simulink model "svpwm_V"  (R2023b)
settings: Solver=FixedStepDiscrete  StartTime=0.0  StopTime=0.05  FixedStep=0.001  MaxStep=0.00001  RelTol=1e-3
libraries: simulink x3
settings Model: Creator=Administrator  LastModifiedBy=LQY
settings SolverCC: AlgebraicLoopSolver=TrustRegion
settings DataIOCC: LimitDataPoints=on  SaveFormat=Array  SignalLoggingSaveFormat=ModelDataLogs  ReturnWorkspaceOutputs=off
settings OptimizationCC: DefaultParameterBehavior=Inlined  UseDivisionForNetSlopeComputation=on  GainParamInheritBuiltInType=on  UseFloatMulNetSlope=on  InlineInvariantSignals=on  PassReuseOutputArgsAs=Individual arguments  ExpressionDepthLimit=2147483647  ZeroExternalMemoryAtStartup=off  ZeroInternalMemoryAtStartup=off  NoFixptDivByZeroProtection=on  EfficientFloat2IntCast=on  LifeSpan=1  OptimizeBlockOrder=speed  DifferentSizesBufferReuse=on  EfficientTunableParamExpr=on
settings DebuggingCC: SaveWithParameterizedLinksMsg=none  UnderspecifiedInitializationDetection=Classic  MergeDetectMultiDrivingBlocksExec=none  SignalResolutionControl=TryResolveAllWithWarning  SolverPrmCheckMsg=warning  MultiTaskDSMMsg=warning  MultiTaskCondExecSysMsg=none  ParameterPrecisionLossMsg=none  ParameterTunabilityLossMsg=error  FcnCallInpInsideContextMsg=warning  UnconnectedInputMsg=warning  UnconnectedOutputMsg=warning  UnconnectedLineMsg=warning  StateNameClashWarn=warning  SFUnexpectedBacktrackingDiag=warning  SFNoUnconditionalDefaultTransitionDiag=warning  SFExecutionAtInitializationDiag=none  ArithmeticOperatorsInVariantConditions=warning
settings HardwareCC: ProdLongLongMode=on
settings ModelReferenceCC: PropagateSignalLabelsOutOfModel=off
settings SFSimCC: SimUseLocalCustomCode=off  MATLABDynamicMemAlloc=off  CustomCodeUndefinedFunction=UseInterfaceOnly
settings RTWCC: Description=Embedded Coder  SystemTargetFile=ert.tlc  GenCodeOnly=on  TemplateMakefile=ert_default_tmf  RTWUseLocalCustomCode=off
settings CodeAppCC: ForceParamTrailComments=on  IgnoreCustomStorageClasses=off  OperatorAnnotations=on  SimulinkDataObjDesc=on  SFDataObjDesc=on  CustomSymbolStrGlobalVar=rt$N$M  CustomSymbolStrType=$N$M  CustomSymbolStrFcn=$N$M$F  CustomSymbolStrMacro=$N$M  InsertBlockDesc=on
settings ERTTargetCC: GenerateSampleERTMain=on  IncludeMdlTerminateFcn=off  CombineSignalStateStructs=on  SuppressErrorStatus=on  SupportAbsoluteTime=off  SupportComplex=off  InlinedParameterPlacement=NonHierarchical  ERTCustomFileTemplate=example_file_process.tlc  ERTFilePackagingFormat=CompactWithDataFile
settings ConfigComp: CovMetricSettings=dw  CovSaveCumulativeToWorkspaceVar=on  CovSaveSingleToWorkspaceVar=on  CovExternalEMLEnable=off

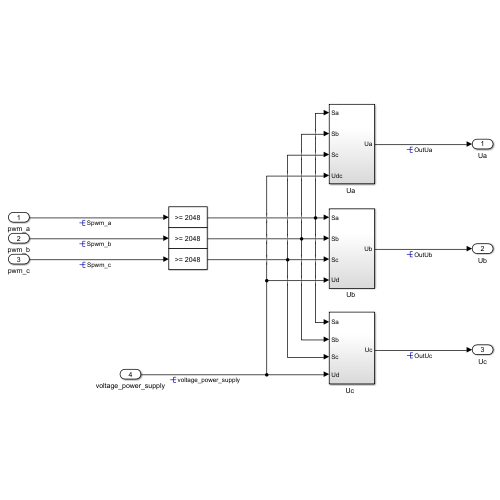
[thumbnail: Simulink's stored preview of the top-level diagram]
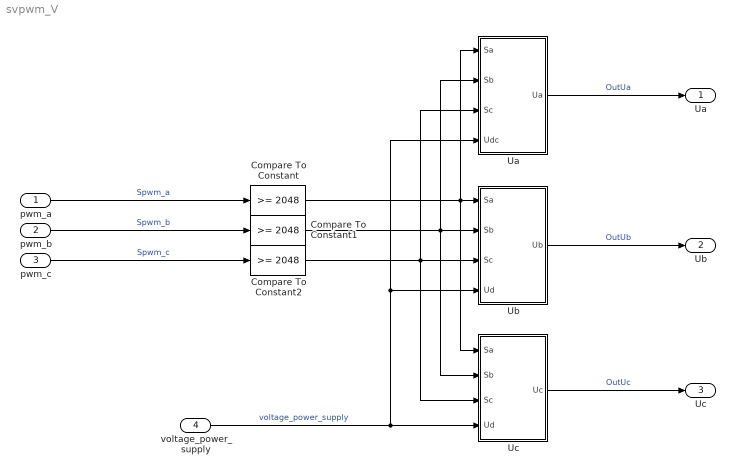
== system svpwm_V ==
  pwm_a : Inport
  pwm_b : Inport  Port=2
  pwm_c : Inport  Port=3
  voltage_power_supply : Inport  Port=4
  Compare To Constant : simulink/Logic and Bit Operations/Compare To Constant  relop=>=  const=2048  OutDataTypeStr=boolean
  Compare To Constant1 : simulink/Logic and Bit Operations/Compare To Constant  relop=>=  const=2048  OutDataTypeStr=boolean
  Compare To Constant2 : simulink/Logic and Bit Operations/Compare To Constant  relop=>=  const=2048  OutDataTypeStr=boolean
  "Ua " : Subsystem
  "Ub " : Subsystem
  "Uc  " : Subsystem
  Ua : Outport
  Ub : Outport  Port=2
  Uc : Outport  Port=3
  wires:
  Compare To Constant/1 -> "Uc  "/1("Sa "), "Ua "/1(Sa), "Ub "/1(Sa)
  Compare To Constant1/1 -> "Uc  "/2(Sb), "Ua "/2(Sb), "Ub "/2(Sb)
  Compare To Constant2/1 -> "Uc  "/3(Sc), "Ua "/3(Sc), "Ub "/3(Sc)
  "Ua "/1(Ua) -> Ua/1  "OutUa"
  "Ub "/1(Ub) -> Ub/1  "OutUb"
  "Uc  "/1(Uc) -> Uc/1  "OutUc"
  voltage_power_supply/1 -> "Uc  "/4(Ud), "Ua "/4(Udc), "Ub "/4(Ud)  "voltage_power_supply"
  pwm_a/1 -> Compare To Constant/1  "Spwm_a"
  pwm_b/1 -> Compare To Constant1/1  "Spwm_b"
  pwm_c/1 -> Compare To Constant2/1  "Spwm_c"

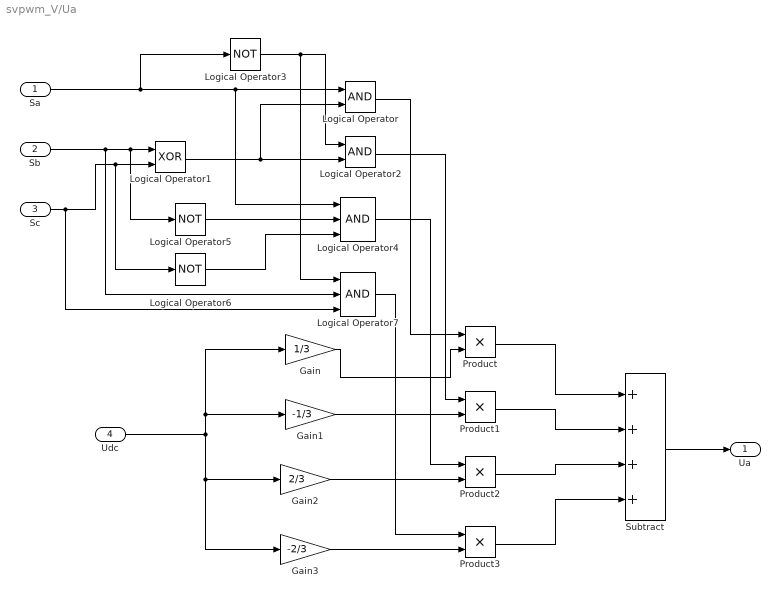
== system svpwm_V/Ua  ==
  Sa : Inport
  Sb : Inport  Port=2
  Sc : Inport  Port=3
  Udc : Inport  Port=4
  Gain : Gain  Gain=1/3
  Gain1 : Gain  Gain=-1/3
  Gain2 : Gain  Gain=2/3
  Gain3 : Gain  Gain=-2/3
  Logical Operator : Logic  AllPortsSameDT=off  OutDataTypeStr=boolean
  Logical Operator1 : Logic  Operator=XOR  AllPortsSameDT=off  OutDataTypeStr=boolean
  Logical Operator2 : Logic  AllPortsSameDT=off  OutDataTypeStr=boolean
  Logical Operator3 : Logic  Operator=NOT  AllPortsSameDT=off  OutDataTypeStr=boolean
  Logical Operator4 : Logic  Inputs=3  AllPortsSameDT=off  OutDataTypeStr=boolean
  Logical Operator5 : Logic  Operator=NOT  AllPortsSameDT=off  OutDataTypeStr=boolean
  Logical Operator6 : Logic  Operator=NOT  AllPortsSameDT=off  OutDataTypeStr=boolean
  Logical Operator7 : Logic  Inputs=3  AllPortsSameDT=off  OutDataTypeStr=boolean
  Product{,1..3} (4 alike) : Product  RndMeth=Zero
  Subtract : Sum  Inputs=++++
  Ua : Outport
  wires:
  Udc/1 -> Gain3/1, Gain2/1, Gain1/1, Gain/1
  Gain/1 -> Product/2
  Gain1/1 -> Product1/2
  Gain2/1 -> Product2/2
  Gain3/1 -> Product3/2
  Product/1 -> Subtract/1
  Product1/1 -> Subtract/2
  Product2/1 -> Subtract/3
  Product3/1 -> Subtract/4
  Subtract/1 -> Ua/1
  Logical Operator/1 -> Product/1
  Sa/1 -> Logical Operator4/1, Logical Operator/1, Logical Operator3/1
  Sb/1 -> Logical Operator7/2, Logical Operator5/1, Logical Operator1/1
  Sc/1 -> Logical Operator7/3, Logical Operator6/1, Logical Operator1/2
  Logical Operator1/1 -> Logical Operator/2, Logical Operator2/2
  Logical Operator2/1 -> Product1/1
  Logical Operator3/1 -> Logical Operator2/1, Logical Operator7/1
  Logical Operator4/1 -> Product2/1
  Logical Operator5/1 -> Logical Operator4/2
  Logical Operator6/1 -> Logical Operator4/3
  Logical Operator7/1 -> Product3/1

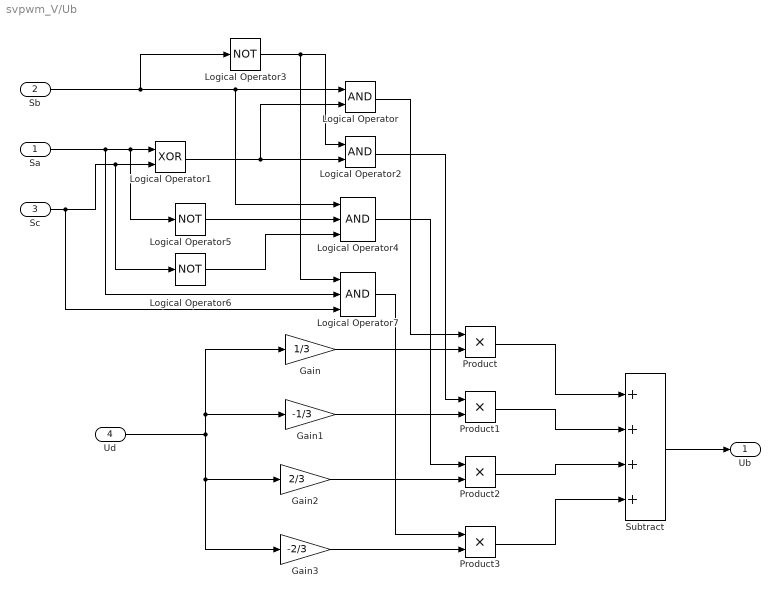
== system svpwm_V/Ub  ==
  Sa : Inport
  Sb : Inport  Port=2
  Sc : Inport  Port=3
  Ud : Inport  Port=4
  Gain : Gain  Gain=1/3
  Gain1 : Gain  Gain=-1/3
  Gain2 : Gain  Gain=2/3
  Gain3 : Gain  Gain=-2/3
  Logical Operator : Logic  AllPortsSameDT=off  OutDataTypeStr=boolean
  Logical Operator1 : Logic  Operator=XOR  AllPortsSameDT=off  OutDataTypeStr=boolean
  Logical Operator2 : Logic  AllPortsSameDT=off  OutDataTypeStr=boolean
  Logical Operator3 : Logic  Operator=NOT  AllPortsSameDT=off  OutDataTypeStr=boolean
  Logical Operator4 : Logic  Inputs=3  AllPortsSameDT=off  OutDataTypeStr=boolean
  Logical Operator5 : Logic  Operator=NOT  AllPortsSameDT=off  OutDataTypeStr=boolean
  Logical Operator6 : Logic  Operator=NOT  AllPortsSameDT=off  OutDataTypeStr=boolean
  Logical Operator7 : Logic  Inputs=3  AllPortsSameDT=off  OutDataTypeStr=boolean
  Product{,1..3} (4 alike) : Product  RndMeth=Zero
  Subtract : Sum  Inputs=++++
  Ub : Outport
  wires:
  Ud/1 -> Gain3/1, Gain2/1, Gain1/1, Gain/1
  Gain/1 -> Product/2
  Gain1/1 -> Product1/2
  Gain2/1 -> Product2/2
  Gain3/1 -> Product3/2
  Product/1 -> Subtract/1
  Product1/1 -> Subtract/2
  Product2/1 -> Subtract/3
  Product3/1 -> Subtract/4
  Subtract/1 -> Ub/1
  Logical Operator/1 -> Product/1
  Sb/1 -> Logical Operator4/1, Logical Operator/1, Logical Operator3/1
  Sa/1 -> Logical Operator7/2, Logical Operator5/1, Logical Operator1/1
  Sc/1 -> Logical Operator7/3, Logical Operator6/1, Logical Operator1/2
  Logical Operator1/1 -> Logical Operator/2, Logical Operator2/2
  Logical Operator2/1 -> Product1/1
  Logical Operator3/1 -> Logical Operator2/1, Logical Operator7/1
  Logical Operator4/1 -> Product2/1
  Logical Operator5/1 -> Logical Operator4/2
  Logical Operator6/1 -> Logical Operator4/3
  Logical Operator7/1 -> Product3/1

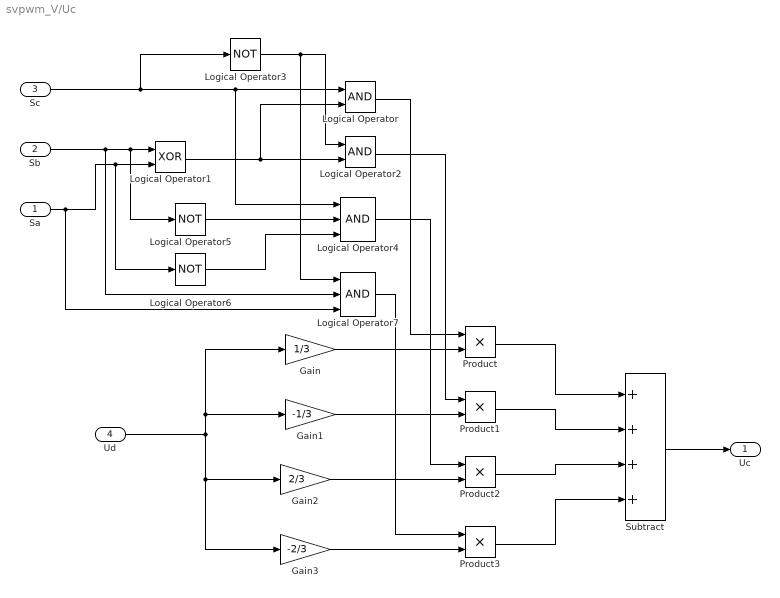
== system svpwm_V/Uc   ==
  "Sa " : Inport
  Sb : Inport  Port=2
  Sc : Inport  Port=3
  Ud : Inport  Port=4
  Gain : Gain  Gain=1/3
  Gain1 : Gain  Gain=-1/3
  Gain2 : Gain  Gain=2/3
  Gain3 : Gain  Gain=-2/3
  Logical Operator : Logic  AllPortsSameDT=off  OutDataTypeStr=boolean
  Logical Operator1 : Logic  Operator=XOR  AllPortsSameDT=off  OutDataTypeStr=boolean
  Logical Operator2 : Logic  AllPortsSameDT=off  OutDataTypeStr=boolean
  Logical Operator3 : Logic  Operator=NOT  AllPortsSameDT=off  OutDataTypeStr=boolean
  Logical Operator4 : Logic  Inputs=3  AllPortsSameDT=off  OutDataTypeStr=boolean
  Logical Operator5 : Logic  Operator=NOT  AllPortsSameDT=off  OutDataTypeStr=boolean
  Logical Operator6 : Logic  Operator=NOT  AllPortsSameDT=off  OutDataTypeStr=boolean
  Logical Operator7 : Logic  Inputs=3  AllPortsSameDT=off  OutDataTypeStr=boolean
  Product{,1..3} (4 alike) : Product  RndMeth=Zero
  Subtract : Sum  Inputs=++++
  Uc : Outport
  wires:
  Ud/1 -> Gain3/1, Gain2/1, Gain1/1, Gain/1
  Gain/1 -> Product/2
  Gain1/1 -> Product1/2
  Gain2/1 -> Product2/2
  Gain3/1 -> Product3/2
  Product/1 -> Subtract/1
  Product1/1 -> Subtract/2
  Product2/1 -> Subtract/3
  Product3/1 -> Subtract/4
  Subtract/1 -> Uc/1
  Logical Operator/1 -> Product/1
  Sc/1 -> Logical Operator4/1, Logical Operator/1, Logical Operator3/1
  Sb/1 -> Logical Operator7/2, Logical Operator5/1, Logical Operator1/1
  "Sa "/1 -> Logical Operator7/3, Logical Operator6/1, Logical Operator1/2
  Logical Operator1/1 -> Logical Operator/2, Logical Operator2/2
  Logical Operator2/1 -> Product1/1
  Logical Operator3/1 -> Logical Operator2/1, Logical Operator7/1
  Logical Operator4/1 -> Product2/1
  Logical Operator5/1 -> Logical Operator4/2
  Logical Operator6/1 -> Logical Operator4/3
  Logical Operator7/1 -> Product3/1
